simulink model "EX5_zadanie1"  (R2023b)
settings: Solver=FixedStepDiscrete  StartTime=0.0  StopTime=0  RelTol=1e-3
libraries: CPOiS_SourcesSinks x12, CPOiS_DataManipulation x4, CPOiS_DataManipulation_IntroduceNoise x2, CPOiS_Filters x2
settings Model: Creator=alyskawa  LastModifiedBy=alyskawa

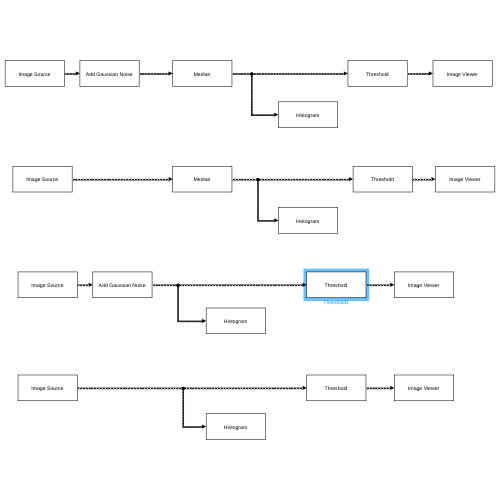
[thumbnail: Simulink's stored preview of the top-level diagram]
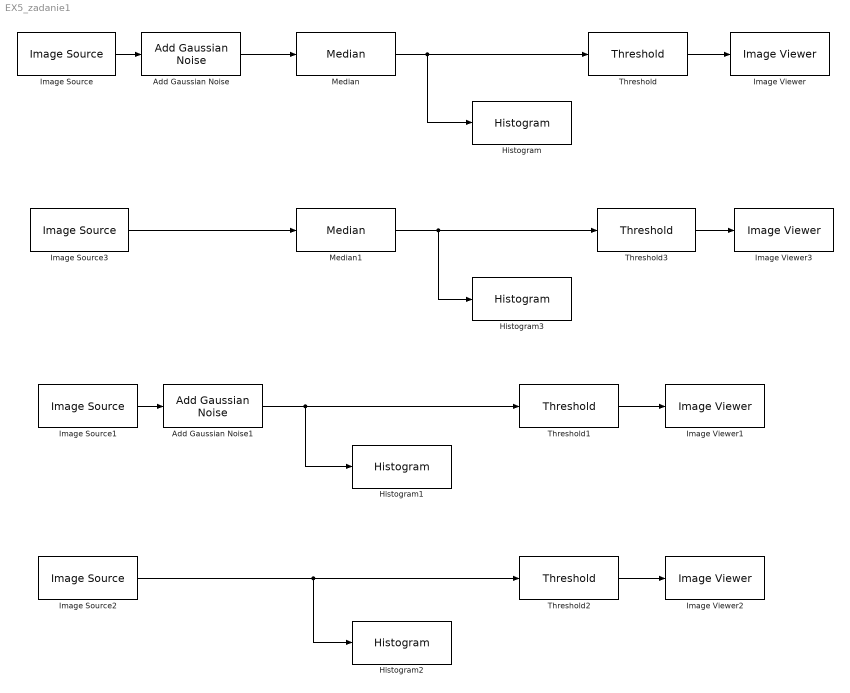
== system EX5_zadanie1 ==
  Add Gaussian Noise : CPOiS_DataManipulation_IntroduceNoise/Add Gaussian Noise  Mean=0  Variance=1
      settings: SourceProductName=CPOiS - Digital image and signal processing
  Add Gaussian Noise1 : CPOiS_DataManipulation_IntroduceNoise/Add Gaussian Noise  Mean=0  Variance=1
      settings: SourceProductName=CPOiS - Digital image and signal processing
  Histogram{,1..3} (4 alike) : CPOiS_SourcesSinks/Histogram
      settings: SourceProductName=CPOiS - Digital image and signal processing
  Image Source{,1..3} (4 alike) : CPOiS_SourcesSinks/Image Source  FileSelection=ball.png
      settings: SourceProductName=CPOiS - Digital image and signal processing
  Image Viewer{,1..3} (4 alike) : CPOiS_SourcesSinks/Image Viewer
      settings: SourceProductName=CPOiS - Digital image and signal processing
  Median : CPOiS_Filters/Median  MaskSize=3 x 3
      settings: SourceProductName=CPOiS - Digital image and signal processing
  Median1 : CPOiS_Filters/Median  MaskSize=3 x 3
      settings: SourceProductName=CPOiS - Digital image and signal processing
  Threshold : CPOiS_DataManipulation/Threshold  Threshold=70
      settings: SourceProductName=CPOiS - Digital image and signal processing
  Threshold1 : CPOiS_DataManipulation/Threshold  Threshold=70
      settings: SourceProductName=CPOiS - Digital image and signal processing
  Threshold2 : CPOiS_DataManipulation/Threshold  Threshold=90
      settings: SourceProductName=CPOiS - Digital image and signal processing
  Threshold3 : CPOiS_DataManipulation/Threshold  Threshold=90
      settings: SourceProductName=CPOiS - Digital image and signal processing
  wires:
  Threshold3/1 -> Image Viewer3/1
  Median/1 -> Histogram/1, Threshold/1
  Image Source3/1 -> Median1/1
  Threshold1/1 -> Image Viewer1/1
  Add Gaussian Noise1/1 -> Histogram1/1, Threshold1/1
  Image Source/1 -> Add Gaussian Noise/1
  Image Source2/1 -> Threshold2/1, Histogram2/1
  Image Source1/1 -> Add Gaussian Noise1/1
  Median1/1 -> Threshold3/1, Histogram3/1
  Threshold/1 -> Image Viewer/1
  Add Gaussian Noise/1 -> Median/1
  Threshold2/1 -> Image Viewer2/1
